simulink model "rootlocus"  (R2019b)
settings: Solver=VariableStepAuto  StartTime=0.0  StopTime=30  RelTol=1e-3
values from neighbouring files (symbols this model uses):
  d_den = [L*Je L*b+R*Je+kt*ke R*b]    [SystemModel.m]
  d_num = [L*r R*r]    [SystemModel.m]
  dt = 0.2    [SystemModel.m]
  fd = fd_vec(1)    [SystemModel.m]
  gain = double(solve(k*abs(((s+a_choice)/(s+b_pole))*((t)/(a*s^3+b*s^2+c*s+d)))==1,k))    [SystemModel.m]
  lag_den = [1 d]    [SystemModel.m]
  lag_num = [1 c]    [SystemModel.m]
  lead_den = [1 b_pole]    [SystemModel.m]
  lead_num = [1 a_choice]    [SystemModel.m]
  p_den = [L*Je L*b+R*Je+kt*ke R*b]    [SystemModel.m]
  p_num = [kt]    [SystemModel.m]
  t_den = [1 tau]    [SystemModel.m]
  t_num = [tau]    [SystemModel.m]
  time = dist_time(1)    [SystemModel.m]
undefined symbols (not defined in the file or in its folder): ref
settings Model: Creator=keato  LastModifiedBy=keato

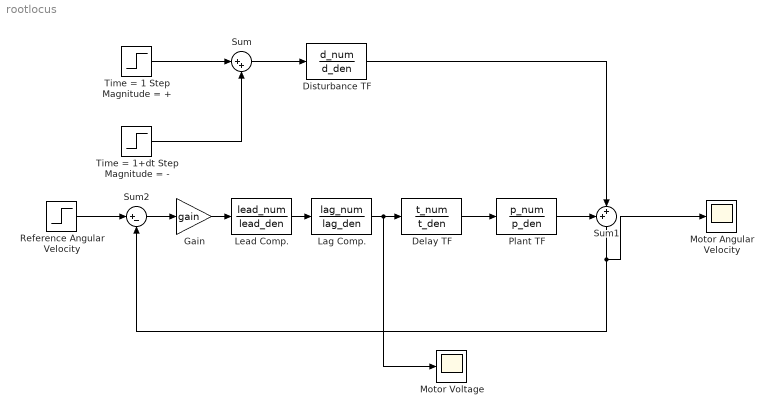
== system rootlocus ==
  Delay TF : TransferFcn  Numerator=t_num  Denominator=t_den
  Disturbance TF : TransferFcn  Numerator=d_num  Denominator=d_den
  Gain : Gain  Gain=gain
  Lag Comp. : TransferFcn  Numerator=lag_num  Denominator=lag_den
  Lead Comp. : TransferFcn  Numerator=lead_num  Denominator=lead_den
  Motor Angular Velocity : Scope
  Motor Voltage : Scope
  Plant TF : TransferFcn  Numerator=p_num  Denominator=p_den
  Reference Angular Velocity : Step  After=ref  SampleTime=0
  Sum : Sum  Inputs=|++
  Sum1 : Sum  Inputs=++|
  Sum2 : Sum  Inputs=|+-
  Time = 1 Step Magnitude = + : Step  Time=time  After=fd  SampleTime=0
  Time = 1+dt Step Magnitude = - : Step  Time=time+dt  After=-fd  SampleTime=0
  wires:
  Sum1/1 -> Sum2/2, Motor Angular Velocity/1
  Plant TF/1 -> Sum1/1
  Sum/1 -> Disturbance TF/1
  Time = 1 Step Magnitude = +/1 -> Sum/1
  Delay TF/1 -> Plant TF/1
  Time = 1+dt Step Magnitude = -/1 -> Sum/2
  Disturbance TF/1 -> Sum1/2
  Reference Angular Velocity/1 -> Sum2/1
  Sum2/1 -> Gain/1
  Gain/1 -> Lead Comp./1
  Lead Comp./1 -> Lag Comp./1
  Lag Comp./1 -> Motor Voltage/1, Delay TF/1
